simulink model "rlKinovaBallBalance_lags"  (R2024a)
settings: Solver=ode15s  StartTime=0.0  StopTime=inf  MaxStep=0.005  RelTol=1e-4  AbsTol=1e-4
values from neighbouring files (symbols this model uses):
  abs_max_torque_U = [6, 0.70, 2.12, 0.505]    [kinova_params.m]
  g = 3.71    [kinova_params.m]
  max_angular_vel = 2.0    (= 2)    [kinova_params.m]
  max_linear_vel = 0.6    [kinova_params.m]
  max_torque = [1.6; 0.6; 0.9; 0.5]    [kinova_params.m]
  max_torque_PD = [2.5; 0.6; 0.6; 0.3]    [kinova_params.m]
  R1_q0 = 0    [kinova_params.m]
  R2_q0 = deg2rad(20)    [kinova_params.m]
  R3_q0 = 0    [kinova_params.m]
  R4_q0 = deg2rad(135)    [kinova_params.m]
  R5_q0 = 0    [kinova_params.m]
  R6_q0 = deg2rad(-65)    [kinova_params.m]
  R7_q0 = deg2rad(-90)    [kinova_params.m]
  rlEpisodeFinalTime = 21    [kinova_params.m]
  rlStartTime = 0    [kinova_params.m]
  rlTimeStep = 0.01    [kinova_params.m]
  U0 = [-5.75, 0.10, -1.3, 0.0]    [kinova_params.m]
undefined symbols (not defined in the file or in its folder): Control, fluent0, L1, L2, L3, LS1, LS3, plate, R1, R2, R3, Rover, rover_path, RS1, RS3, Ts, vessel, X, Y, Z
libraries: sm_lib x251, nesl_utility x110, fl_lib x85, nesl_utility_internal x34, sdl_lib x20, simulink x16, ee_lib x10, mars_rover_lib x6, slpidlib x2, batteryecm_lib x2, robotalgslib x1, rllib x1
(part 1 of 13)
settings Model: VariantFading=off  Creator=cosorio  LastModifiedBy=dika
settings SolverCC: AlgebraicLoopSolver=TrustRegion  MaxZcPerStep=1
settings DataIOCC: DSMLogging=off
settings OptimizationCC: ReuseModelBlockBuffer=off
settings DebuggingCC: UnconnectedInputMsg=warning  UnconnectedOutputMsg=warning  UnconnectedLineMsg=warning
settings ModelReferenceCC: EnableRefExpFcnMdlSchedulingChecks=on
settings RTWCC: GPUComputeCapability=3.5  DLArmComputeVersion=19.05
settings ExplorerConfigSet: InternalSimMechanicsExplorerSettings="<ExplorerConfiguration><canonicalview>default</canonicalview><AnimationSetting><BasePlaybackSpeed>1.0</BasePlaybackSpeed><PlaybackSpeedFactor>1.0</PlaybackSpeedFactor></AnimationSetting><TilePanel><TileInfo><Tiles Columns=\"1\" Count=\"1\" Rows=\"1\"><Column Weight=\"1\"/><Row Weight=\"1\"/><Tile Height=\"1\" Width=\"1\" X=\"0\" Y=\"0\"/></Tiles></TileInfo><SceneInfo><SceneViewer><BGColor><R>1</R><G>1</G><B>1</B></BGColor><Camera><DoPerspective>off</DoPerspective><Position><X>0.835449044511457073</X><Y>-0.495506913595096854</Y><Z>0.970261214764596258</Z></Position><Center><X>0.258098775321831175</X><Y>0.0818433555945289881</Y><Z>0.392910945574970416</Z></Center><Up><X>-0.408248290463863073</X><Y>0.408248290463863073</Y><Z>0.816496580927726145</Z></Up><ViewLimDist>1</ViewLimDist><YLim>0.340419242978096004</YLim><XLim>0.488995507299471222</XLim></Camera></SceneViewer></SceneInfo></TilePanel><MechEditorPanel><Cameras/><GfxPanelCameraMap/><VideoCreator><PlaybackSpeedRatio>1.0</PlaybackSpeedRatio><FrameRate>30</FrameRate><VideoFormat>Motion JPEG AVI</VideoFormat><FrameSize>auto</FrameSize></VideoCreator></MechEditorPanel></ExplorerConfiguration>"

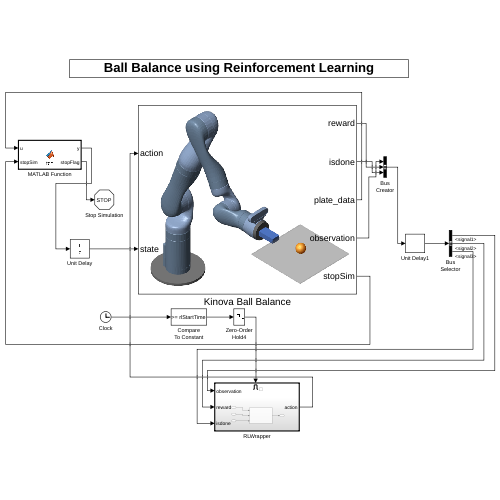
[thumbnail: Simulink's stored preview of the top-level diagram]
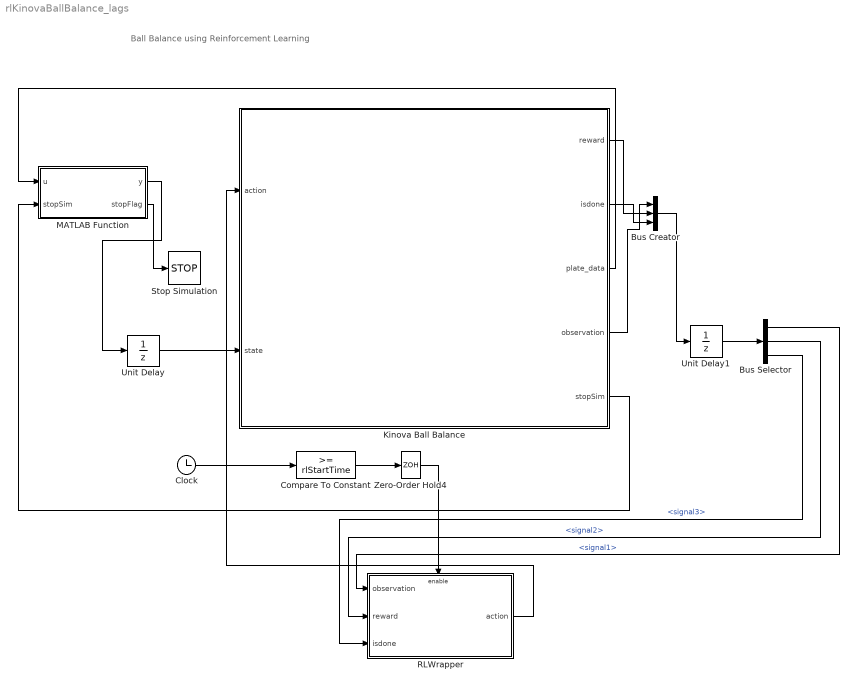
== system rlKinovaBallBalance_lags ==
  note: Ball Balance using Reinforcement Learning
  Bus Creator : BusCreator  Inputs=3
  Bus Selector : BusSelector  OutputSignals=signal1,signal2,signal3
  Clock : Clock
  Compare To Constant : simulink/Logic and Bit Operations/Compare To Constant  relop=>=  const=rlStartTime  OutDataTypeStr=boolean
  Kinova Ball Balance : Subsystem
      mask Display: image('$imagefile'); % Use "Edit Image" on toolstrip to change.
  MATLAB Function : MATLAB Function  TreatAsAtomicUnit=on
  RLWrapper : Subsystem  TreatAsAtomicUnit=on
  Stop Simulation : Stop
  Unit Delay : UnitDelay  SampleTime=-1  HasFrameUpgradeWarning=on
  Unit Delay1 : UnitDelay  SampleTime=-1  HasFrameUpgradeWarning=on
  Zero-Order Hold4 : ZeroOrderHold  SampleTime=Ts
  wires:
  MATLAB Function/1(y) -> Unit Delay/1
  Unit Delay/1 -> Kinova Ball Balance/2(state)
  Kinova Ball Balance/3(plate_data) -> MATLAB Function/1(u)
  Kinova Ball Balance/1(reward) -> Bus Creator/2
  Kinova Ball Balance/2(isdone) -> Bus Creator/3
  Bus Creator/1 -> Unit Delay1/1
  Unit Delay1/1 -> Bus Selector/1
  Kinova Ball Balance/4(observation) -> Bus Creator/1
  Bus Selector/2 -> RLWrapper/2(reward)  "<signal2>"
  Bus Selector/1 -> RLWrapper/1(observation)  "<signal1>"
  Bus Selector/3 -> RLWrapper/3(isdone)  "<signal3>"
  RLWrapper/1(action) -> Kinova Ball Balance/1(action)
  Compare To Constant/1 -> Zero-Order Hold4/1
  Clock/1 -> Compare To Constant/1
  Kinova Ball Balance/5(stopSim) -> MATLAB Function/2(stopSim)
  Zero-Order Hold4/1 -> RLWrapper/Enable
  MATLAB Function/2(stopFlag) -> Stop Simulation/1

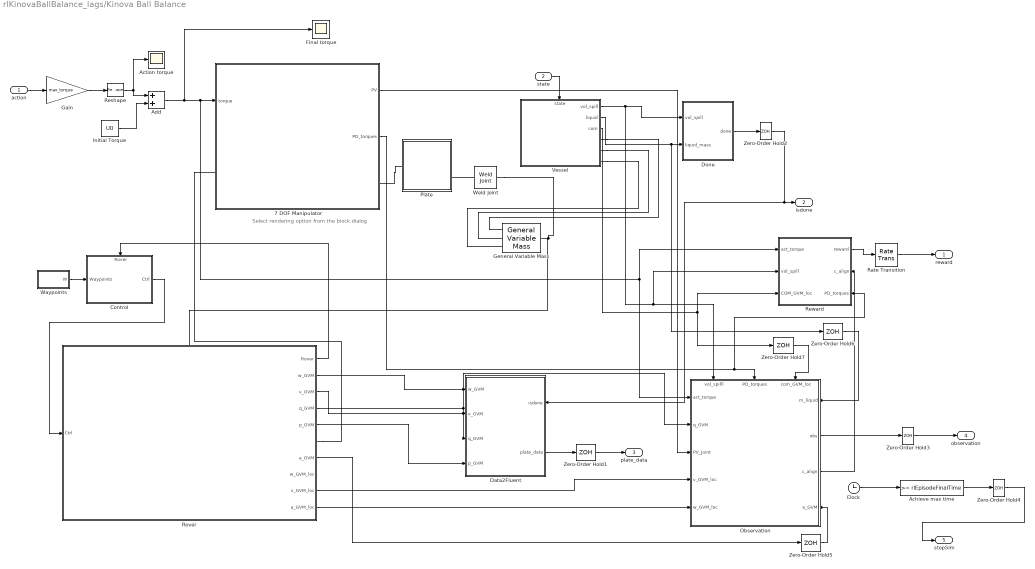
== system rlKinovaBallBalance_lags/Kinova Ball Balance ==
  note: Select rendering option from the block dialog
  action : Inport
  state : Inport  Port=2
  7 DOF Manipulator : Subsystem  mask{VChoice=3D Mesh}
      mask prompts: VChoice "Visualization"
      mask init:
      | choice = get_param(gcb,'VChoice');
      | vssBlk = bdroot + "/Kinova Ball Balance/7 DOF Manipulator" + ...
      |    ["/base_link/Base Link";
      |     "/Shoulder_Link/Shoulder Link";
      |     "/HalfArm1_Link/HalfArm1 Link";
      |     "/HalfArm2_Link/HalfArm2 Link";
      |     "/ForeArm_Link/ForeArm Link";
      |     "/Wrist1_Link/Wrist1 Link";
      |     "/Wrist2_Link/Wrist2 Link";
      |     "/Bracelet_Link/Bracelet Link"];
      | oldVariant = get_param(gcb,'LabelModeActiveChoice');
      | for ct = 1:numel(vssBlk)
      |     if strcmp(choice,'None')
      |         % turn off simscape visualization
      |         set_param(vssBlk(ct), 'LabelModeActiveChoice', 'Choice');
      |         set_param(bdroot, 'SimMechanicsOpenEditorOnUpdate', 'off');
      |     else
      |         % turn on simscape visualization
      |         set_param(vssBlk(ct), 'LabelModeActiveChoice', 'Choice_1');
      |         set_param(bdroot, 'SimMechanicsOpenEditorOnUpdate', 'on');
      |     end
      | end
      mask TypeOptions VChoice: None | 3D Mesh
      mask DialogControl DescGroupVar Prompt: Rendering
      mask DialogControl DescTextVar Prompt: Select options to visualize the robot. The 3D Mesh option requires the Robotics System Toolbox Robot Library Data support package.
      mask DialogControl ParameterGroupVar Prompt: Rendering options
      mask Display: image('$imagefile'); % Use "Edit Image" on toolstrip to change.
  Achieve max time : simulink/Logic and Bit Operations/Compare To Constant  relop=>=  const=rlEpisodeFinalTime  OutDataTypeStr=boolean
  Action torque : Scope
  Add : Sum
  Clock : Clock
  Control : Subsystem
      settings: PortSchema="{\"entries\":[{\"content\":{\"sides\":[{\"content\":{\"connectorIds\":[\"In1\"]},\"type\":\"ConnectorPlacement.EquallySpacedRectSide\",\"uuid\":\"c3d7e194-f80c-4e55-926d-d58bd075eaae\"},{\"content\":{\"connectorIds\":[\"Out1\"],\"side\":\"RIGHT\"},\"type\":\"ConnectorPlacement.EquallySpacedRectSide\",\"uuid\":\"f7d0fe5b-9aee-419d-9958-60715756a35f\"},{\"content\":{\"connectorIds\":[\"In2\"],\"side\":\"TOP\"},\"type\":\"ConnectorPlacement.EquallySpacedRectSide\",\"uuid\":\"f91288f6-db9b-4528-8971-65b8d23b6b9e\"},{\"content\":{\"side\":\"BOTTOM\"},\"type\":\"ConnectorPlacement.EquallySpacedRectSide\",\"uuid\":\"aa6c6625-5d2c-4cfa-81dd-42b85ff12eb6\"}]},\"type\":\"ConnectorPlacement.EquallySpacedConnector\",\"uuid\":\"3d017957-8f60-4a25-bb87-fd20ede06be0\"}],\"packageUris\":[\"http://schema.mathworks.com/mf0/Connector/R2020b\"],\"version\":\"1.0\"}"
  Data2Fluent : Subsystem
      settings: PortSchema="{\"entries\":[{\"content\":{\"sides\":[{\"content\":{\"connectorIds\":[\"In1\",\"In2\",\"In3\",\"In4\"]},\"type\":\"ConnectorPlacement.EquallySpacedRectSide\",\"uuid\":\"d2580b95-1100-4ac1-85be-11deaa0122b6\"},{\"content\":{\"connectorIds\":[\"In5\",\"Out1\"],\"side\":\"RIGHT\"},\"type\":\"ConnectorPlacement.EquallySpacedRectSide\",\"uuid\":\"70e7c1d6-5559-4655-a09c-42417fa5168e\"},{\"content\":{\"side\":\"TOP\"},\"type\":\"ConnectorPlacement.EquallySpacedRectSide\",\"uuid\":\"be848a5e-034e-48a0-9929-21b8a0be8f3f\"}]},\"type\":\"ConnectorPlacement.EquallySpacedConnector\",\"uuid\":\"450ed5cd-5d65-4ed6-b2f4-ea103b2a194f\"}],\"packageUris\":[\"http://schema.mathworks.com/mf0/Connector/R2020b\"],\"version\":\"1.0\"}"
  Done : Subsystem
  Final torque : Scope
  Gain : Gain  Gain=max_torque
  General Variable Mass : sm_lib/Body Elements/Variable Mass/General Variable Mass  VariableInertiaType=Custom  MassType=TimeVarying  Mass=1  MassUnits=kg  CenterOfMassType=TimeVarying  CenterOfMass=[0 0 0]  CenterOfMassUnits=m  InertiaMatrixType=TimeVarying  MomentsOfInertia=[1 1 1]  MomentsOfInertiaUnits=kg*m^2  ProductsOfInertia=[0 0 0]  ProductsOfInertiaUnits=kg*m^2  GraphicType=Marker  MarkerShape=Sphere  MarkerSize=100  GraphicVisPropType=SimpleVisualProperties  GraphicDiffuseColor=[0.5 0.5 0.5]  GraphicOpacity=1  GraphicSpecularColor=[0.5 0.5 0.5 1.0]  GraphicAmbientColor=[0.15 0.15 0.15 1.0]  GraphicEmissiveColor=[0.0 0.0 0.0 1.0]  GraphicShininess=75
  Initial Torque : Constant  Value=U0
  Observation : Subsystem
      settings: PortSchema="{\"entries\":[{\"content\":{\"sides\":[{\"content\":{\"connectorIds\":[\"In1\",\"In2\",\"In3\",\"In4\",\"In5\"]},\"type\":\"ConnectorPlacement.EquallySpacedRectSide\",\"uuid\":\"1f819b26-4f65-41ef-a298-effbe2270ef5\"},{\"content\":{\"connectorIds\":[\"In9\",\"Out1\",\"Out2\",\"In10\"],\"side\":\"RIGHT\"},\"type\":\"ConnectorPlacement.EquallySpacedRectSide\",\"uuid\":\"491918ce-fc7c-4684-8246-c6be896d1069\"},{\"content\":{\"connectorIds\":[\"In6\",\"In7\",\"In8\"],\"side\":\"TOP\"},\"type\":\"ConnectorPlacement.EquallySpacedRectSide\",\"uuid\":\"2c72369d-314e-4a7a-93e9-42ede2c72e3e\"},{\"content\":{\"side\":\"BOTTOM\"},\"type\":\"ConnectorPlacement.EquallySpacedRectSide\",\"uuid\":\"f3733c5f-ece3-4511-b18e-584e8db17e04\"}]},\"type\":\"ConnectorPlacement.EquallySpacedConnector\",\"uuid\":\"9fa8ee02-96e6-4ca3-a042-fc1037b88a21\"}],\"packageUris\":[\"http://schema.mathworks.com/mf0/Connector/R2020b\"],\"version\":\"1.0\"}"
  Plate : Subsystem
      mask Display: image('$imagefile'); % Use "Edit Image" on toolstrip to change.
  Rate Transition : RateTransition  OutPortSampleTime=Ts
  Reshape : Reshape  OutputDimensionality=Row vector (2-D)
  Reward : Subsystem
      settings: PortSchema="{\"entries\":[{\"content\":{\"sides\":[{\"content\":{\"connectorIds\":[\"In1\",\"In2\",\"In3\"]},\"type\":\"ConnectorPlacement.EquallySpacedRectSide\",\"uuid\":\"5d933a9d-95d3-47ea-9901-687451c9fbea\"},{\"content\":{\"connectorIds\":[\"Out1\",\"In4\",\"In5\"],\"side\":\"RIGHT\"},\"type\":\"ConnectorPlacement.EquallySpacedRectSide\",\"uuid\":\"29a52886-19a3-4b66-bd74-438fafa7a07e\"},{\"content\":{\"side\":\"TOP\"},\"type\":\"ConnectorPlacement.EquallySpacedRectSide\",\"uuid\":\"3fc8db25-df22-4142-aace-f1d33f79f87b\"}]},\"type\":\"ConnectorPlacement.EquallySpacedConnector\",\"uuid\":\"35028655-dfec-48a2-9708-f2ca1e0329cc\"}],\"packageUris\":[\"http://schema.mathworks.com/mf0/Connector/R2020b\"],\"version\":\"1.0\"}"
  Rover : Subsystem
      settings: PortSchema="{\"entries\":[{\"content\":{\"sides\":[{\"content\":{\"connectorIds\":[\"In1\"]},\"type\":\"ConnectorPlacement.EquallySpacedRectSide\",\"uuid\":\"f99998cd-7f44-4958-986a-883545f054e6\"},{\"content\":{\"connectorIds\":[\"Out1\",\"Out2\",\"Out3\",\"Out4\",\"Out5\",\"RConn1\",\"Out6\",\"Out7\",\"Out8\",\"Out9\"],\"side\":\"RIGHT\"},\"type\":\"ConnectorPlacement.EquallySpacedRectSide\",\"uuid\":\"f32f7cef-c0c0-4695-a0b9-122721d5e398\"},{\"content\":{\"connectorIds\":[\"LConn1\"],\"side\":\"TOP\"},\"type\":\"ConnectorPlacement.EquallySpacedRectSide\",\"uuid\":\"7344a25a-a782-4a10-9f2c-7810aaabe583\"}]},\"type\":\"ConnectorPlacement.EquallySpacedConnector\",\"uuid\":\"21be1294-6a1a-40f2-9693-1f444d473d1d\"}],\"packageUris\":[\"http://schema.mathworks.com/mf0/Connector/R2020b\"],\"version\":\"1.0\"}"
      mask Display: image('mars_rover_terrain_chassis.png');
  Vessel : Subsystem
      settings: PortSchema="{\"entries\":[{\"content\":{\"sides\":[{\"content\":{},\"type\":\"ConnectorPlacement.EquallySpacedRectSide\",\"uuid\":\"dcdc7885-492c-498f-a442-6424ac696a17\"},{\"content\":{\"connectorIds\":[\"Out1\",\"Out2\",\"Out3\",\"RConn1\",\"RConn2\",\"RConn3\"],\"side\":\"RIGHT\"},\"type\":\"ConnectorPlacement.EquallySpacedRectSide\",\"uuid\":\"323b1566-cd85-443c-b64d-37bc7cbbf4f4\"},{\"content\":{\"connectorIds\":[\"In1\"],\"side\":\"TOP\"},\"type\":\"ConnectorPlacement.EquallySpacedRectSide\",\"uuid\":\"18ea813b-2836-4610-9c93-f73d3123e495\"},{\"content\":{\"side\":\"BOTTOM\"},\"type\":\"ConnectorPlacement.EquallySpacedRectSide\",\"uuid\":\"bc1a7a95-2321-49a3-b611-36fcfe7a8e53\"}]},\"type\":\"ConnectorPlacement.EquallySpacedConnector\",\"uuid\":\"32ac73cf-4f09-4885-b08e-9ed6f73651df\"}],\"packageUris\":[\"http://schema.mathworks.com/mf0/Connector/R2020b\"],\"version\":\"1.0\"}"
  Waypoints : Subsystem
      mask Display:
      | px = evalin('base','rover_path.x');
      | py = evalin('base','rover_path.y');
      | plot(px,py)
  Weld Joint : sm_lib/Joints/Weld Joint  JointMode=Normal  CompositeWrenchDir=FollowerOnBase  CompositeWrenchFrame=BaseFrame  SenseConstraintForce=off  SenseConstraintTorque=off  SenseTotalForce=off  SenseTotalTorque=off
  Zero-Order Hold{1..7} (7 alike) : ZeroOrderHold  SampleTime=Ts
  reward : Outport
  isdone : Outport  Port=2
  plate_data : Outport  Port=3
  observation : Outport  Port=4
  stopSim : Outport  Port=5
  wires:
  state/1 -> Vessel/1(state)
  7 DOF Manipulator/1(PV) -> Observation/3(PV_Joint)
  Zero-Order Hold1/1 -> plate_data/1
  Waypoints/1(W) -> Control/1(Waypoints)
  Control/1(Ctrl) -> Rover/1(Ctrl)
  Rover/1(Rover) -> Control/2(Rover)
  Reward/1(reward) -> Rate Transition/1
  Data2Fluent/1(plate_data) -> Zero-Order Hold1/1
  Observation/1(obs) -> Zero-Order Hold3/1
  Rate Transition/1 -> reward/1
  action/1 -> Gain/1
  Done/1(done) -> Zero-Order Hold2/1
  Zero-Order Hold2/1 -> isdone/1, Data2Fluent/5(isdone)
  Gain/1 -> Reshape/1
  Reshape/1 -> Add/1, Action torque/1
  Initial Torque/1 -> Add/2
  Vessel/3(com) -> Zero-Order Hold7/1, Reward/3(COM_GVM_loc)
  Zero-Order Hold3/1 -> observation/1
  Rover/5(p_GVM) -> Data2Fluent/4(p_GVM)
  Rover/4(q_GVM) -> Data2Fluent/3(q_GVM), Observation/2(q_GVM)
  Rover/3(v_GVM) -> Data2Fluent/2(v_GVM)
  Rover/2(w_GVM) -> Data2Fluent/1(w_GVM)
  Vessel/2(liquid) -> Zero-Order Hold6/1, Done/2(liquid_mass)
  Vessel/1(vol_spill) -> Reward/2(vol_spill), Observation/6(vol_spilll), Done/1(vol_spill)
  Clock/1 -> Achieve max time/1
  Achieve max time/1 -> Zero-Order Hold4/1
  Zero-Order Hold4/1 -> stopSim/1
  Rover/6(a_GVM) -> Zero-Order Hold5/1
  Zero-Order Hold5/1 -> Observation/10(a_GVM)
  Zero-Order Hold6/1 -> Observation/9(m_liquid)
  Zero-Order Hold7/1 -> Observation/8(com_GVM_loc)
  Observation/2(c_align) -> Reward/4(c_align)
  Add/1 -> Final torque/1, Observation/1(act_torque), Reward/1(act_torque), 7 DOF Manipulator/1(torque)
  7 DOF Manipulator/2(PD_torques) -> Reward/5(PD_torques), Observation/7(PD_torques)
  Rover/8(v_GVM_loc) -> Observation/4(v_GVM_loc)
  Rover/9(a_GVM_loc) -> Observation/5(w_GVM_loc)
  connections:
  Rover/RConn1 -- 7 DOF Manipulator/LConn1
  Vessel/RConn3 -- General Variable Mass/LConn3
  Weld Joint/RConn1 -- Rover/LConn1 -- General Variable Mass/RConn1
  Vessel/RConn2 -- General Variable Mass/LConn2
  Vessel/RConn1 -- General Variable Mass/LConn1
  Weld Joint/LConn1 -- Plate/LConn2
  7 DOF Manipulator/RConn1 -- Plate/RConn1

== system rlKinovaBallBalance_lags/RLWrapper ==
  observation : Inport
  reward : Inport  Port=2
  isdone : Inport  Port=3
  Enable : EnablePort
  RL Agent : rllib/RL Agent  Agent=agentObj  ExternalActionAsInput=off  ProvideLastAction=off  ProvideCumRwd=off  TreatAsDirectFeedthrough=on  UseStrictObservationDataTypes=off
  action : Outport
  wires:
  isdone/1 -> RL Agent/3
  observation/1 -> RL Agent/1
  reward/1 -> RL Agent/2
  RL Agent/1 -> action/1

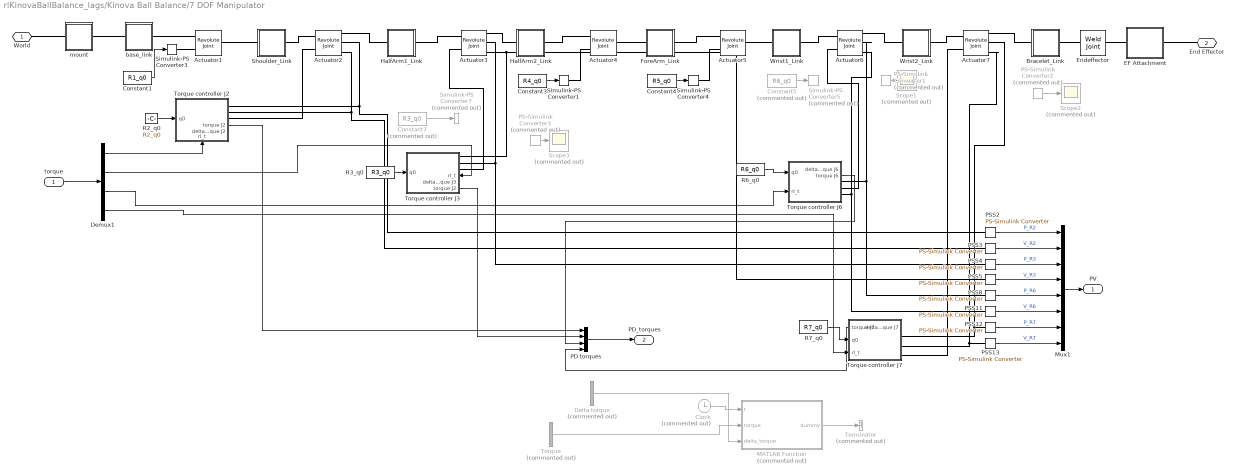
== system rlKinovaBallBalance_lags/Kinova Ball Balance/7 DOF Manipulator ==
  torque : Inport
  Actuator1 : sm_lib/Joints/Revolute Joint  JointMode=Normal  CompositeWrenchDir=FollowerOnBase  CompositeWrenchFrame=BaseFrame  SenseConstraintForce=off  SenseConstraintTorque=off  SenseTotalForce=off  SenseTotalTorque=off  PositionTargetSpecify=on  PositionTargetPriority=High  PositionTargetValue=R1_q0  PositionTargetValueUnits=rad  VelocityTargetSpecify=off  VelocityTargetPriority=High  VelocityTargetValue=0  VelocityTargetValueUnits=deg/s  EquilibriumPosition=0  EquilibriumPositionUnits=deg  SpringStiffness=0  SpringStiffnessUnits=N*m/deg  DampingCoefficient=0  DampingCoefficientUnits=m^2*kg/s/rad  LowerLimitSpecify=off  LowerLimitBound=-90  LowerLimitBoundUnits=deg  LowerLimitStiffness=1e4  LowerLimitStiffnessUnits=N*m/deg  LowerLimitDamping=10  LowerLimitDampingUnits=N*m/(deg/s)  LowerLimitTransitionRegionWidth=0.1  LowerLimitTransitionRegionWidthUnits=deg  UpperLimitSpecify=off  UpperLimitBound=90  UpperLimitBoundUnits=deg  UpperLimitStiffness=1e4  UpperLimitStiffnessUnits=N*m/deg  UpperLimitDamping=10  UpperLimitDampingUnits=N*m/(deg/s)  UpperLimitTransitionRegionWidth=0.1  UpperLimitTransitionRegionWidthUnits=deg  TorqueActuationMode=ComputedTorque  MotionActuationMode=InputMotion  SensePosition=off  SenseVelocity=off  SenseAcceleration=off  SenseTorqueForce=off  SenseLowerLimitTorqueForce=off  SenseUpperLimitTorqueForce=off
  Actuator2 : sm_lib/Joints/Revolute Joint  JointMode=Normal  CompositeWrenchDir=FollowerOnBase  CompositeWrenchFrame=BaseFrame  SenseConstraintForce=off  SenseConstraintTorque=off  SenseTotalForce=off  SenseTotalTorque=off  PositionTargetSpecify=on  PositionTargetPriority=High  PositionTargetValue=R2_q0  PositionTargetValueUnits=rad  VelocityTargetSpecify=off  VelocityTargetPriority=High  VelocityTargetValue=0  VelocityTargetValueUnits=deg/s  EquilibriumPosition=0  EquilibriumPositionUnits=deg  SpringStiffness=50  SpringStiffnessUnits=N*m/rad  DampingCoefficient=5  DampingCoefficientUnits=N*m*s/rad  LowerLimitSpecify=on  LowerLimitBound=-2.2  LowerLimitBoundUnits=rad  LowerLimitStiffness=1e4  LowerLimitStiffnessUnits=N*m/deg  LowerLimitDamping=10  LowerLimitDampingUnits=N*m/(deg/s)  LowerLimitTransitionRegionWidth=0.1  LowerLimitTransitionRegionWidthUnits=deg  UpperLimitSpecify=on  UpperLimitBound=2.2  UpperLimitBoundUnits=rad  UpperLimitStiffness=1e4  UpperLimitStiffnessUnits=N*m/deg  UpperLimitDamping=10  UpperLimitDampingUnits=N*m/(deg/s)  UpperLimitTransitionRegionWidth=0.1  UpperLimitTransitionRegionWidthUnits=deg  TorqueActuationMode=InputTorque  MotionActuationMode=ComputedMotion  SensePosition=on  SenseVelocity=on  SenseAcceleration=off  SenseTorqueForce=off  SenseLowerLimitTorqueForce=off  SenseUpperLimitTorqueForce=off
  Actuator3 : sm_lib/Joints/Revolute Joint  JointMode=Normal  CompositeWrenchDir=FollowerOnBase  CompositeWrenchFrame=BaseFrame  SenseConstraintForce=off  SenseConstraintTorque=off  SenseTotalForce=off  SenseTotalTorque=off  PositionTargetSpecify=on  PositionTargetPriority=High  PositionTargetValue=R3_q0  PositionTargetValueUnits=rad  VelocityTargetSpecify=off  VelocityTargetPriority=High  VelocityTargetValue=0  VelocityTargetValueUnits=deg/s  EquilibriumPosition=0  EquilibriumPositionUnits=deg  SpringStiffness=50  SpringStiffnessUnits=N*m/rad  DampingCoefficient=5  DampingCoefficientUnits=N*m*s/rad  LowerLimitSpecify=off  LowerLimitBound=-90  LowerLimitBoundUnits=deg  LowerLimitStiffness=1e4  LowerLimitStiffnessUnits=N*m/deg  LowerLimitDamping=10  LowerLimitDampingUnits=N*m/(deg/s)  LowerLimitTransitionRegionWidth=0.1  LowerLimitTransitionRegionWidthUnits=deg  UpperLimitSpecify=off  UpperLimitBound=90  UpperLimitBoundUnits=deg  UpperLimitStiffness=1e4  UpperLimitStiffnessUnits=N*m/deg  UpperLimitDamping=10  UpperLimitDampingUnits=N*m/(deg/s)  UpperLimitTransitionRegionWidth=0.1  UpperLimitTransitionRegionWidthUnits=deg  TorqueActuationMode=InputTorque  MotionActuationMode=ComputedMotion  SensePosition=on  SenseVelocity=on  SenseAcceleration=off  SenseTorqueForce=off  SenseLowerLimitTorqueForce=off  SenseUpperLimitTorqueForce=off
  Actuator4 : sm_lib/Joints/Revolute Joint  JointMode=Normal  CompositeWrenchDir=FollowerOnBase  CompositeWrenchFrame=BaseFrame  SenseConstraintForce=off  SenseConstraintTorque=off  SenseTotalForce=off  SenseTotalTorque=off  PositionTargetSpecify=on  PositionTargetPriority=High  PositionTargetValue=R4_q0  PositionTargetValueUnits=rad  VelocityTargetSpecify=off  VelocityTargetPriority=High  VelocityTargetValue=0  VelocityTargetValueUnits=deg/s  EquilibriumPosition=0  EquilibriumPositionUnits=deg  SpringStiffness=0  SpringStiffnessUnits=N*m/deg  DampingCoefficient=0  DampingCoefficientUnits=m^2*kg/s/rad  LowerLimitSpecify=on  LowerLimitBound=-2.5656  LowerLimitBoundUnits=rad  LowerLimitStiffness=1e4  LowerLimitStiffnessUnits=N*m/deg  LowerLimitDamping=10  LowerLimitDampingUnits=N*m/(deg/s)  LowerLimitTransitionRegionWidth=0.1  LowerLimitTransitionRegionWidthUnits=deg  UpperLimitSpecify=on  UpperLimitBound=2.5656  UpperLimitBoundUnits=rad  UpperLimitStiffness=1e4  UpperLimitStiffnessUnits=N*m/deg  UpperLimitDamping=10  UpperLimitDampingUnits=N*m/(deg/s)  UpperLimitTransitionRegionWidth=0.1  UpperLimitTransitionRegionWidthUnits=deg  TorqueActuationMode=ComputedTorque  MotionActuationMode=InputMotion  SensePosition=off  SenseVelocity=off  SenseAcceleration=off  SenseTorqueForce=off  SenseLowerLimitTorqueForce=off  SenseUpperLimitTorqueForce=off
  Actuator5 : sm_lib/Joints/Revolute Joint  JointMode=Normal  CompositeWrenchDir=FollowerOnBase  CompositeWrenchFrame=BaseFrame  SenseConstraintForce=off  SenseConstraintTorque=off  SenseTotalForce=off  SenseTotalTorque=off  PositionTargetSpecify=on  PositionTargetPriority=High  PositionTargetValue=R5_q0  PositionTargetValueUnits=rad  VelocityTargetSpecify=off  VelocityTargetPriority=High  VelocityTargetValue=0  VelocityTargetValueUnits=deg/s  EquilibriumPosition=0  EquilibriumPositionUnits=deg  SpringStiffness=0  SpringStiffnessUnits=N*m/deg  DampingCoefficient=0  DampingCoefficientUnits=m^2*kg/s/rad  LowerLimitSpecify=off  LowerLimitBound=-90  LowerLimitBoundUnits=deg  LowerLimitStiffness=1e4  LowerLimitStiffnessUnits=N*m/deg  LowerLimitDamping=10  LowerLimitDampingUnits=N*m/(deg/s)  LowerLimitTransitionRegionWidth=0.1  LowerLimitTransitionRegionWidthUnits=deg  UpperLimitSpecify=off  UpperLimitBound=90  UpperLimitBoundUnits=deg  UpperLimitStiffness=1e4  UpperLimitStiffnessUnits=N*m/deg  UpperLimitDamping=10  UpperLimitDampingUnits=N*m/(deg/s)  UpperLimitTransitionRegionWidth=0.1  UpperLimitTransitionRegionWidthUnits=deg  TorqueActuationMode=ComputedTorque  MotionActuationMode=InputMotion  SensePosition=off  SenseVelocity=off  SenseAcceleration=off  SenseTorqueForce=off  SenseLowerLimitTorqueForce=off  SenseUpperLimitTorqueForce=off
  Actuator6 : sm_lib/Joints/Revolute Joint  JointMode=Normal  CompositeWrenchDir=FollowerOnBase  CompositeWrenchFrame=BaseFrame  SenseConstraintForce=off  SenseConstraintTorque=off  SenseTotalForce=off  SenseTotalTorque=off  PositionTargetSpecify=on  PositionTargetPriority=High  PositionTargetValue=R6_q0  PositionTargetValueUnits=rad  VelocityTargetSpecify=off  VelocityTargetPriority=High  VelocityTargetValue=0  VelocityTargetValueUnits=deg/s  EquilibriumPosition=0  EquilibriumPositionUnits=deg  SpringStiffness=0  SpringStiffnessUnits=N*m/deg  DampingCoefficient=0  DampingCoefficientUnits=m^2*kg/s/rad  LowerLimitSpecify=on  LowerLimitBound=-2.05  LowerLimitBoundUnits=rad  LowerLimitStiffness=1e4  LowerLimitStiffnessUnits=N*m/deg  LowerLimitDamping=10  LowerLimitDampingUnits=N*m/(deg/s)  LowerLimitTransitionRegionWidth=0.1  LowerLimitTransitionRegionWidthUnits=deg  UpperLimitSpecify=on  UpperLimitBound=2.05  UpperLimitBoundUnits=rad  UpperLimitStiffness=1e4  UpperLimitStiffnessUnits=N*m/deg  UpperLimitDamping=10  UpperLimitDampingUnits=N*m/(deg/s)  UpperLimitTransitionRegionWidth=0.1  UpperLimitTransitionRegionWidthUnits=deg  TorqueActuationMode=InputTorque  MotionActuationMode=ComputedMotion  SensePosition=on  SenseVelocity=on  SenseAcceleration=off  SenseTorqueForce=off  SenseLowerLimitTorqueForce=off  SenseUpperLimitTorqueForce=off
  Actuator7 : sm_lib/Joints/Revolute Joint  JointMode=Normal  CompositeWrenchDir=FollowerOnBase  CompositeWrenchFrame=BaseFrame  SenseConstraintForce=off  SenseConstraintTorque=off  SenseTotalForce=off  SenseTotalTorque=off  PositionTargetSpecify=on  PositionTargetPriority=High  PositionTargetValue=R7_q0  PositionTargetValueUnits=rad  VelocityTargetSpecify=off  VelocityTargetPriority=High  VelocityTargetValue=0  VelocityTargetValueUnits=deg/s  EquilibriumPosition=0  EquilibriumPositionUnits=deg  SpringStiffness=0  SpringStiffnessUnits=N*m/deg  DampingCoefficient=0  DampingCoefficientUnits=m^2*kg/s/rad  LowerLimitSpecify=off  LowerLimitBound=-90  LowerLimitBoundUnits=deg  LowerLimitStiffness=1e4  LowerLimitStiffnessUnits=N*m/deg  LowerLimitDamping=10  LowerLimitDampingUnits=N*m/(deg/s)  LowerLimitTransitionRegionWidth=0.1  LowerLimitTransitionRegionWidthUnits=deg  UpperLimitSpecify=off  UpperLimitBound=90  UpperLimitBoundUnits=deg  UpperLimitStiffness=1e4  UpperLimitStiffnessUnits=N*m/deg  UpperLimitDamping=10  UpperLimitDampingUnits=N*m/(deg/s)  UpperLimitTransitionRegionWidth=0.1  UpperLimitTransitionRegionWidthUnits=deg  TorqueActuationMode=InputTorque  MotionActuationMode=ComputedMotion  SensePosition=on  SenseVelocity=on  SenseAcceleration=off  SenseTorqueForce=off  SenseLowerLimitTorqueForce=off  SenseUpperLimitTorqueForce=off
  Bracelet_Link : Subsystem
  Clock : Clock  Commented=on
  Constant1 : Constant  Value=R1_q0
  Constant3 : Constant  Value=R4_q0
  Constant4 : Constant  Value=R5_q0
  Constant5 : Constant  Commented=on  Value=R6_q0
  Constant7 : Constant  Commented=on  Value=R3_q0
  Delta torque : Mux  Commented=on
  Demux1 : Demux
  EF Attachment : Subsystem
  Endeffector : sm_lib/Joints/Weld Joint  JointMode=Normal  CompositeWrenchDir=FollowerOnBase  CompositeWrenchFrame=BaseFrame  SenseConstraintForce=off  SenseConstraintTorque=off  SenseTotalForce=off  SenseTotalTorque=off
  ForeArm_Link : Subsystem
  HalfArm1_Link : Subsystem
  HalfArm2_Link : Subsystem
  MATLAB Function : MATLAB Function  Commented=on  TreatAsAtomicUnit=on
  Mux1 : Mux  Inputs=8
  PD torques : Mux
  PS-Simulink Converter1 : nesl_utility/PS-Simulink Converter  Commented=on  PhysicalDomain=network_engine_domain  SubClassName=ps_output  LeftPortType=input  RightPortType=output  PseudoPeriodic=off  Frequencies=[]  VectorFormat=inherit  Unit=inherit  AffineConversion=off
  PS-Simulink Converter2 : nesl_utility/PS-Simulink Converter  Commented=on  PhysicalDomain=network_engine_domain  SubClassName=ps_output  LeftPortType=input  RightPortType=output  PseudoPeriodic=off  Frequencies=[]  VectorFormat=inherit  Unit=inherit  AffineConversion=off
  PS-Simulink Converter3 : nesl_utility/PS-Simulink Converter  Commented=on  PhysicalDomain=network_engine_domain  SubClassName=ps_output  LeftPortType=input  RightPortType=output  PseudoPeriodic=off  Frequencies=[]  VectorFormat=inherit  Unit=inherit  AffineConversion=off
  PSS{3,5,11,13} (4 alike) : nesl_utility_internal/PS-Simulink Converter  PhysicalDomain=network_engine_domain  SubClassName=ps_output  LeftPortType=input  RightPortType=output  PseudoPeriodic=off  Frequencies=[]  VectorFormat=1-D array  Unit=rad/s  AffineConversion=off
  PSS{2,4,8,12} (4 alike) : nesl_utility_internal/PS-Simulink Converter  PhysicalDomain=network_engine_domain  SubClassName=ps_output  LeftPortType=input  RightPortType=output  PseudoPeriodic=off  Frequencies=[]  VectorFormat=1-D array  Unit=rad  AffineConversion=off
  R2_q0 : Constant  Value=R2_q0
  R3_q0 : Constant  Value=R3_q0
  R6_q0 : Constant  Value=R6_q0
  R7_q0 : Constant  Value=R7_q0
  Scope1 : Scope  Commented=on
  Scope2 : Scope  Commented=on
  Scope3 : Scope  Commented=on
  Shoulder_Link : Subsystem
  Simulink-PS Converter1 : nesl_utility_internal/Simulink-PS Converter  PhysicalDomain=network_engine_domain  SubClassName=ps_input  LeftPortType=input  RightPortType=output  PseudoPeriodic=off  Frequencies=[]  NoiseDistribution=none  NoiseParameters=[]  Unit=1  AffineConversion=off  FilteringAndDerivatives=provide  SimscapeFilterOrder=1  InputFilterTimeConstant=0.001  UdotUserProvided=0
  Simulink-PS Converter3 : nesl_utility_internal/Simulink-PS Converter  PhysicalDomain=network_engine_domain  SubClassName=ps_input  LeftPortType=input  RightPortType=output  PseudoPeriodic=off  Frequencies=[]  NoiseDistribution=none  NoiseParameters=[]  Unit=1  AffineConversion=off  FilteringAndDerivatives=provide  SimscapeFilterOrder=1  InputFilterTimeConstant=0.001  UdotUserProvided=0
  Simulink-PS Converter4 : nesl_utility_internal/Simulink-PS Converter  PhysicalDomain=network_engine_domain  SubClassName=ps_input  LeftPortType=input  RightPortType=output  PseudoPeriodic=off  Frequencies=[]  NoiseDistribution=none  NoiseParameters=[]  Unit=1  AffineConversion=off  FilteringAndDerivatives=provide  SimscapeFilterOrder=1  InputFilterTimeConstant=0.001  UdotUserProvided=0
  Simulink-PS Converter5 : nesl_utility_internal/Simulink-PS Converter  Commented=on  PhysicalDomain=network_engine_domain  SubClassName=ps_input  LeftPortType=input  RightPortType=output  PseudoPeriodic=off  Frequencies=[]  NoiseDistribution=none  NoiseParameters=[]  Unit=1  AffineConversion=off  FilteringAndDerivatives=provide  SimscapeFilterOrder=1  InputFilterTimeConstant=0.001  UdotUserProvided=0
  Simulink-PS Converter7 : nesl_utility_internal/Simulink-PS Converter  Commented=on  PhysicalDomain=network_engine_domain  SubClassName=ps_input  LeftPortType=input  RightPortType=output  PseudoPeriodic=off  Frequencies=[]  NoiseDistribution=none  NoiseParameters=[]  Unit=1  AffineConversion=off  FilteringAndDerivatives=provide  SimscapeFilterOrder=1  InputFilterTimeConstant=0.001  UdotUserProvided=0
  Terminator : Terminator  Commented=on
  Torque : Mux  Commented=on
  Torque controller J2 : Subsystem
      settings: PortSchema="{\"entries\":[{\"content\":{\"sides\":[{\"content\":{\"connectorIds\":[\"In1\"]},\"type\":\"ConnectorPlacement.EquallySpacedRectSide\",\"uuid\":\"095988aa-34ff-41fa-a977-f46d39e23b2a\"},{\"content\":{\"connectorIds\":[\"RConn1\",\"RConn2\",\"RConn3\",\"Out1\",\"Out2\"],\"side\":\"RIGHT\"},\"type\":\"ConnectorPlacement.EquallySpacedRectSide\",\"uuid\":\"f68620a5-2921-48f0-865e-8506c5ca8f7b\"},{\"content\":{\"side\":\"TOP\"},\"type\":\"ConnectorPlacement.EquallySpacedRectSide\",\"uuid\":\"eeebf0d3-0cb1-47e5-8559-57fe666debe6\"},{\"content\":{\"connectorIds\":[\"In2\"],\"side\":\"BOTTOM\"},\"type\":\"ConnectorPlacement.EquallySpacedRectSide\",\"uuid\":\"535c76d7-2393-4bc1-beaf-0c16d2a56ade\"}]},\"type\":\"ConnectorPlacement.EquallySpacedConnector\",\"uuid\":\"bdca3cdb-44ac-4f4f-9fc0-a63e5a64f5ef\"}],\"packageUris\":[\"http://schema.mathworks.com/mf0/Connector/R2020b\"],\"version\":\"1.0\"}"
  Torque controller J3 : Subsystem
      settings: PortSchema="{\"entries\":[{\"content\":{\"sides\":[{\"content\":{\"connectorIds\":[\"In1\"]},\"type\":\"ConnectorPlacement.EquallySpacedRectSide\",\"uuid\":\"095988aa-34ff-41fa-a977-f46d39e23b2a\"},{\"content\":{\"connectorIds\":[\"RConn1\",\"RConn2\",\"RConn3\",\"In2\",\"Out1\",\"Out2\"],\"side\":\"RIGHT\"},\"type\":\"ConnectorPlacement.EquallySpacedRectSide\",\"uuid\":\"f68620a5-2921-48f0-865e-8506c5ca8f7b\"},{\"content\":{\"side\":\"TOP\"},\"type\":\"ConnectorPlacement.EquallySpacedRectSide\",\"uuid\":\"eeebf0d3-0cb1-47e5-8559-57fe666debe6\"}]},\"type\":\"ConnectorPlacement.EquallySpacedConnector\",\"uuid\":\"bdca3cdb-44ac-4f4f-9fc0-a63e5a64f5ef\"}],\"packageUris\":[\"http://schema.mathworks.com/mf0/Connector/R2020b\"],\"version\":\"1.0\"}"
  Torque controller J6 : Subsystem
  Torque controller J7 : Subsystem
      settings: PortSchema="{\"entries\":[{\"content\":{\"sides\":[{\"content\":{\"connectorIds\":[\"Out2\",\"In1\",\"In2\"]},\"type\":\"ConnectorPlacement.EquallySpacedRectSide\",\"uuid\":\"2ba4fbae-ef3a-4af5-8190-ba61f5af81f4\"},{\"content\":{\"connectorIds\":[\"Out1\",\"RConn1\",\"RConn2\",\"RConn3\"],\"side\":\"RIGHT\"},\"type\":\"ConnectorPlacement.EquallySpacedRectSide\",\"uuid\":\"932be769-d022-4bca-b733-10e6d8a94a22\"},{\"content\":{\"side\":\"TOP\"},\"type\":\"ConnectorPlacement.EquallySpacedRectSide\",\"uuid\":\"afed630b-2a44-4167-8319-4873b4e3e0f0\"}]},\"type\":\"ConnectorPlacement.EquallySpacedConnector\",\"uuid\":\"48d452e0-ef32-4a0a-be11-1a1156200253\"}],\"packageUris\":[\"http://schema.mathworks.com/mf0/Connector/R2020b\"],\"version\":\"1.0\"}"
  Wrist1_Link : Subsystem
  Wrist2_Link : Subsystem
  base_link : Subsystem
  mount : Subsystem
  World : PMIOPort  Side=Left
  End Effector : PMIOPort  Port=2  Side=Right
  PV : Outport
  PD_torques : Outport  Port=2
  wires:
  Constant3/1 -> Simulink-PS Converter1/1
  Constant4/1 -> Simulink-PS Converter4/1
  torque/1 -> Demux1/1
  PSS11/1 -> Mux1/6  "V_R6"
  PSS8/1 -> Mux1/5  "P_R6"
  PSS5/1 -> Mux1/4  "V_R3"
  PSS4/1 -> Mux1/3  "P_R3"
  PSS3/1 -> Mux1/2  "V_R2"
  PSS2/1 -> Mux1/1  "P_R2"
  Mux1/1 -> PV/1
  PSS12/1 -> Mux1/7  "P_R7"
  PSS13/1 -> Mux1/8  "V_R7"
  PS-Simulink Converter1/1 -> Scope1/1
  Constant5/1 -> Simulink-PS Converter5/1
  PS-Simulink Converter2/1 -> Scope2/1
  Constant7/1 -> Simulink-PS Converter7/1
  PS-Simulink Converter3/1 -> Scope3/1
  Constant1/1 -> Simulink-PS Converter3/1
  R7_q0/1 -> Torque controller J7/1(q0)
  R3_q0/1 -> Torque controller J3/1(q0)
  R6_q0/1 -> Torque controller J6/1(q0)
  R2_q0/1 -> Torque controller J2/1(q0)
  Demux1/2 -> Torque controller J3/2(rl_t)
  Demux1/3 -> Torque controller J6/2(rl_t)
  Demux1/4 -> Torque controller J7/2(rl_t)
  Demux1/1 -> Torque controller J2/2(rl_t)
  Delta torque/1 -> MATLAB Function/3(delta_torque)
  Torque/1 -> MATLAB Function/2(torque)
  Clock/1 -> MATLAB Function/1(t)
  MATLAB Function/1(dummy) -> Terminator/1
  Torque controller J2/1(torque J2) -> PD torques/1
  Torque controller J3/2(torque J2) -> PD torques/2
  Torque controller J6/2(torque J6) -> PD torques/3
  Torque controller J7/2(torque J7) -> PD torques/4
  PD torques/1 -> PD_torques/1
  connections:
  Actuator1/RConn1 -- Shoulder_Link/LConn1
  Actuator2/RConn1 -- HalfArm1_Link/LConn1
  Actuator1/LConn1 -- base_link/RConn1
  Actuator7/LConn1 -- Wrist2_Link/RConn1
  Actuator3/RConn1 -- HalfArm2_Link/LConn1
  Actuator4/LConn1 -- HalfArm2_Link/RConn1
  Actuator6/LConn1 -- Wrist1_Link/RConn1
  Actuator4/RConn1 -- ForeArm_Link/LConn1
  Actuator3/LConn1 -- HalfArm1_Link/RConn1
  Bracelet_Link/RConn1 -- Endeffector/LConn1
  Actuator5/RConn1 -- Wrist1_Link/LConn1
  Actuator5/LConn1 -- ForeArm_Link/RConn1
  Actuator2/LConn1 -- Shoulder_Link/RConn1
  Actuator6/RConn1 -- Wrist2_Link/LConn1
  Actuator7/RConn1 -- Bracelet_Link/LConn1
  Simulink-PS Converter1/RConn1 -- Actuator4/LConn2
  End Effector/RConn1 -- EF Attachment/RConn1
  EF Attachment/LConn1 -- Endeffector/RConn1
  World/RConn1 -- mount/RConn1
  mount/LConn1 -- base_link/LConn1
  Actuator3/RConn2 -- PSS4/LConn1 -- Torque controller J3/RConn2
  Actuator3/RConn3 -- Torque controller J3/RConn1 -- PSS5/LConn1
  Actuator6/RConn2 -- Torque controller J6/RConn1 -- PSS8/LConn1
  Actuator6/RConn3 -- Torque controller J6/RConn3 -- PSS11/LConn1
  Actuator7/RConn2 -- Torque controller J7/RConn1 -- PSS12/LConn1
  Actuator7/RConn3 -- Torque controller J7/RConn2 -- PSS13/LConn1
  Simulink-PS Converter4/RConn1 -- Actuator5/LConn2
  Actuator2/RConn3 -- PSS3/LConn1 -- Torque controller J2/RConn2
  Actuator2/RConn2 -- Torque controller J2/RConn1 -- PSS2/LConn1
  Simulink-PS Converter3/RConn1 -- Actuator1/LConn2
  Actuator2/LConn2 -- Torque controller J2/RConn3
  Torque controller J3/RConn3 -- Actuator3/LConn2
  Torque controller J6/RConn2 -- Actuator6/LConn2
  Torque controller J7/RConn3 -- Actuator7/LConn2

== system rlKinovaBallBalance_lags/Kinova Ball Balance/Control ==
  Waypoints : Inport
  In Bus Element1 : Inport  Port=2  PortName=Rover  Element=Chassis
  In Bus Element5 : Inport  Port=2  PortName=Rover  Element=Body
  Chassis Control : Subsystem
  Out Bus Element1 : Outport  PortName=Ctrl  Element=Chassis
  wires:
  Waypoints/1 -> Chassis Control/1(Waypoints)
  Chassis Control/1(Ctrl) -> Out Bus Element1/1
  In Bus Element1/1 -> Chassis Control/2(Chassis)
  In Bus Element5/1 -> Chassis Control/3(Body)

== system rlKinovaBallBalance_lags/Kinova Ball Balance/Data2Fluent ==
  w_GVM : Inport
  v_GVM : Inport  Port=2
  q_GVM : Inport  Port=3
  p_GVM : Inport  Port=4
  isdone : Inport  Port=5
  Data Type Conversion : DataTypeConversion  OutDataTypeStr=double  SaturateOnIntegerOverflow=off  RndMeth=Floor
  Demux p : Demux  Outputs=3
  Demux q : Demux
  Demux v : Demux  Outputs=3
  Demux w : Demux  Outputs=3
  Mux : Mux  Inputs=14
  plate_data : Outport
  wires:
  q_GVM/1 -> Demux q/1
  Demux q/4 -> Mux/7  "q4"
  Demux p/1 -> Mux/1  "Px"
  Demux p/2 -> Mux/2  "Py"
  Demux p/3 -> Mux/3  "Pz"
  Demux q/1 -> Mux/4  "q1"
  Demux q/2 -> Mux/5  "q2"
  Demux q/3 -> Mux/6  "q3"
  Demux v/1 -> Mux/8  "vx"
  Demux v/2 -> Mux/9  "vy"
  Demux v/3 -> Mux/10  "vz"
  Mux/1 -> plate_data/1
  Demux w/1 -> Mux/11  "wx"
  Demux w/2 -> Mux/12  "wy"
  Demux w/3 -> Mux/13  "wz"
  isdone/1 -> Data Type Conversion/1
  Data Type Conversion/1 -> Mux/14
  v_GVM/1 -> Demux v/1
  w_GVM/1 -> Demux w/1
  p_GVM/1 -> Demux p/1

== system rlKinovaBallBalance_lags/Kinova Ball Balance/Done ==
  vol_spill : Inport
  liquid_mass : Inport  Port=2
  AND : Logic  IconShape=distinctive  AllPortsSameDT=off  OutDataTypeStr=boolean
  Compare To Constant : simulink/Logic and Bit Operations/Compare To Constant  relop=>  const=0  OutDataTypeStr=boolean
  Compare To Constant1 : simulink/Logic and Bit Operations/Compare To Constant  relop=<  const=fluent0.m*0.7  OutDataTypeStr=boolean
  Compare To Constant2 : simulink/Logic and Bit Operations/Compare To Constant  relop=>=  const=fluent0.m*0.3*0.001  OutDataTypeStr=boolean
  OR : Logic  Operator=OR  IconShape=distinctive  AllPortsSameDT=off  OutDataTypeStr=boolean
  done : Outport
  wires:
  AND/1 -> OR/2
  Compare To Constant1/1 -> AND/1
  Compare To Constant/1 -> AND/2
  liquid_mass/1 -> Compare To Constant/1, Compare To Constant1/1
  OR/1 -> done/1
  vol_spill/1 -> Compare To Constant2/1
  Compare To Constant2/1 -> OR/1

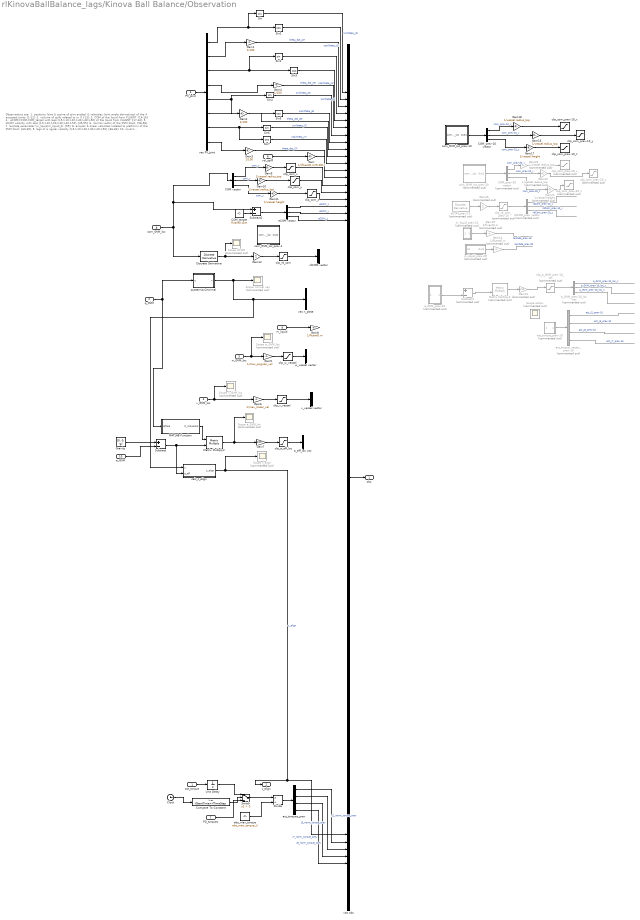
== system rlKinovaBallBalance_lags/Kinova Ball Balance/Observation ==
  note: Observations are:
      | 1. positions (sine & cosine of joint angles) & velocities (joint angle derivatives) of the 4 actuated joints {1-12}
      | 2. volume of spills related to m_0 {13}
      | 3. COM of the liquid from FLUENT {14-16}
      | 4 . eCOM=COM-COM_target with lags [t-5,t-10,t-20,t-30,t-40,t-50] of the liquid from FLUENT {17-34}
      | 5. dCOM velocity with lags [t-5,t-10,t-20,t-30,t-40,t-50] {35-55}
      | 6. normal vector of the GVM block {56-58}
      | 7. lambda parameter (m_liquid/m_liquid_0) {59}
      | 8. angular & linear velocities (related to platform) of the GVM block {60-65}
      | 9. lags of a ngular velocity [t-5,t-10,t-20,t-30,t-40,t-50] {66-83}
      | 10. rover's acceleration related to GVM local system a_eff_loc=quatToR_W2vessel[qPlate](Mars_gravity-a_chassis) {84-86}
      | 11. lags of a_eff_loc [t-5,t-10,t-20,t-30,t-40,t-50] {87-104}
      | 12. c_align = a_GVM / (||a_GVM||+epsilon)*dot*n_plate {105}
      | 13. 1-step lag for torques: act_torque_prev {106-109}
  act_torque : Inport
  q_GVM : Inport  Port=2
  PV_Joint : Inport  Port=3
  v_GVM_loc : Inport  Port=4
  w_GVM_loc : Inport  Port=5
  vol_spilll : Inport  Port=6
  PD_torques : Inport  Port=7
  com_GVM_loc : Inport  Port=8
  m_liquid : Inport  Port=9
  a_GVM : Inport  Port=10
  COM vector : Demux  Outputs=3
  COM_prev-10 vector : Demux  Outputs=3
  COM_prev-20 vector : Demux  Commented=on  Outputs=3
  COM_target : Constant  Value=fluent0.com
  Clock : Clock
  Compare To Constant : simulink/Logic and Bit Operations/Compare To Constant  relop=>=  const=rlStartTime+rlTimeStep  OutDataTypeStr=boolean
  Discrete Derivative : simulink/Discrete/Discrete Derivative  gainval=1.0  ICPrevScaledInput=0.0  OutMin=[]  OutMax=[]  OutDataType=fixdt(1, 16)  OutScaling=2^-10  DoSatur=off
  Divide : Product  Inputs=*/
  Gain : Gain  Gain=1/(fluent0.m*0.001)
  Gain{1..4} (4 alike) : Gain  Gain=1/100
  Gain{9..10,16,18} (4 alike) : Gain  Gain=1/vessel.radius_top
  Gain11 : Gain  Gain=1/vessel.height
  Gain12 : Gain
  Gain13 : Gain  Commented=on  Gain=1/10
  Gain14 : Gain  Commented=on  Gain=1/fluent0.m
  Gain15 : Gain  Commented=on
  Gain17 : Gain  Gain=1/vessel.height
  Gain19 : Gain  Commented=on  Gain=1/fluent0.m
  Gain20 : Gain  Commented=on  Gain=1/vessel.radius_top
  Gain21 : Gain  Commented=on  Gain=1/vessel.height
  Gain22 : Gain  Commented=on  Gain=1/vessel.radius_top
  Gain5 : Gain  Gain=1/max_angular_vel
  Gain6 : Gain  Gain=1/max_linear_vel
  Gain7 : Gain  Gain=1/10
  Gain8 : Gain  Gain=1/fluent0.m
  Gravity : Constant  Value=[0; 0; -g]
  MATLAB Function : MATLAB Function  TreatAsAtomicUnit=on
  Matrix Multiply2 : Product  Multiplication=Matrix(*)
  Matrix Multiply3 : Product  Commented=on  Multiplication=Matrix(*)
  Scope a_GVM_loc : Scope  Commented=on
  Scope action : Scope  Commented=on
  Scope c_align : Scope  Commented=on
  Scope dCOM : Scope  Commented=on
  Scope normal vec : Scope  Commented=on
  Scope v_GVM_loc : Scope  Commented=on
  Scope w_GVM_loc : Scope  Commented=on
  Sin{,1,4,6} (4 alike) : Trigonometry
  Sin{2..3,5,7} (4 alike) : Trigonometry  Operator=cos
  Subtract : Sum  Inputs=+-
  Subtract1 : Sum  Commented=on  Inputs=+-
  Subtract2 : Sum  Inputs=+-
  Switch : Switch  Criteria=u2 > Threshold  ZeroCross=off  SaturateOnIntegerOverflow=off  InputSameDT=off
  Unit Delay : UnitDelay  SampleTime=-1  HasFrameUpgradeWarning=on
  a_GVM_prev-10 : Subsystem  Commented=on
  a_GVM_prev-10_loc vec : Demux  Commented=on  Outputs=3
  a_eff_loc vec : Demux  Outputs=3
  abs_max_torque : Constant  Value=abs_max_torque_U
  act_torque_prev-10 : Subsystem  Commented=on
  act_torque_vector_prev-10 : Demux  Commented=on
  act_torques_prev : Demux
  calc_c_align : MATLAB Function  TreatAsAtomicUnit=on
  clip_a_GVM_prev-10_loc : Saturate  Commented=on  UpperLimit=1  LowerLimit=-1
  clip_a_eff_loc : Saturate  UpperLimit=1  LowerLimit=-1
  clip_com_prev-10_x : Saturate  UpperLimit=1  LowerLimit=-1
  clip_com_prev-10_y : Saturate  UpperLimit=1  LowerLimit=-1
  clip_com_prev-10_z : Saturate  UpperLimit=1  LowerLimit=-1
  clip_com_prev-20_x : Saturate  Commented=on  UpperLimit=1  LowerLimit=-1
  clip_com_prev-20_y : Saturate  Commented=on  UpperLimit=1  LowerLimit=-1
  clip_com_prev-20_z : Saturate  Commented=on  UpperLimit=1  LowerLimit=-1
  clip_com_x : Saturate  UpperLimit=1  LowerLimit=-1
  clip_com_y : Saturate  UpperLimit=1  LowerLimit=-1
  clip_com_z : Saturate  UpperLimit=1  LowerLimit=-1
  clip_rd_com : Saturate  UpperLimit=1  LowerLimit=-1
  clip_rd_com_prev-10 : Saturate  Commented=on  UpperLimit=1  LowerLimit=-1
  clip_v_vessel : Saturate  UpperLimit=1  LowerLimit=-1
  clip_w_vessel : Saturate  UpperLimit=1  LowerLimit=-1
  com_GVM_loc_prev-1 : Subsystem
  com_GVM_loc_prev-10 : Subsystem
  com_GVM_loc_prev-20 : Subsystem  Commented=on
  dCOM_prev-10 : simulink/Discrete/Discrete Derivative  Commented=on  gainval=1.0  ICPrevScaledInput=0.0  OutMin=[]  OutMax=[]  OutDataType=fixdt(1, 16)  OutScaling=2^-10  DoSatur=off
  eCOM vector : Demux  Outputs=3
  m_liquid_prev-10 : Subsystem  Commented=on
  m_liquid_prev-20 : Subsystem  Commented=on
  quaternion2normal : MATLAB Function  TreatAsAtomicUnit=on
  rdCOM vector : Demux  Outputs=3
  rdCOM_prev vector : Demux  Commented=on  Outputs=3
  v_vessel vector : Demux  Outputs=3
  vec PV_Joint : Demux  Outputs=8
  vec n_plate : Demux  Outputs=3
  vec obs : Mux  Inputs=109
  w_vessel vector : Demux  Outputs=3
  obs : Outport
  c_align : Outport  Port=2
  wires:
  PV_Joint/1 -> vec PV_Joint/1
  vec PV_Joint/1 -> Sin/1, Sin2/1
  vec PV_Joint/3 -> Sin1/1, Sin3/1
  vec PV_Joint/4 -> Gain4/1
  Sin/1 -> vec obs/1  "sin(theta_J2)"
  vec obs/1 -> obs/1
  Sin2/1 -> vec obs/2  "cos(theta_J2)"
  Sin1/1 -> vec obs/4  "sin(theta_J3)"
  Sin3/1 -> vec obs/5  "cos(theta_J3)"
  Gain1/1 -> vec obs/3  "theta_dot_J2*"
  vec PV_Joint/6 -> Gain2/1
  vec PV_Joint/8 -> Gain3/1
  Sin6/1 -> vec obs/10  "sin(theta_J7)"
  Sin7/1 -> vec obs/11  "cos(theta_J7)"
  Gain2/1 -> vec obs/9  "theta_dot_J6*"
  Gain3/1 -> vec obs/12  "theta_dot_J7*"
  COM vector/1 -> Gain9/1  "com_x"
  COM vector/2 -> Gain10/1  "com_y"
  COM vector/3 -> Gain11/1  "com_z"
  vol_spilll/1 -> Gain/1
  Gain/1 -> vec obs/13
  w_GVM_loc/1 -> Scope w_GVM_loc/1, Gain5/1
  v_GVM_loc/1 -> Scope v_GVM_loc/1, Gain6/1
  a_GVM/1 -> Subtract/2
  MATLAB Function/1(R_W2vessel) -> Matrix Multiply2/1
  Subtract/1 -> calc_c_align/2(a_eff), Matrix Multiply2/2
  Matrix Multiply2/1 -> Scope a_GVM_loc/1, Gain7/1
  Discrete Derivative/1 -> Scope dCOM/1, Gain12/1
  clip_rd_com/1 -> rdCOM vector/1
  Gain7/1 -> clip_a_eff_loc/1
  m_liquid/1 -> Gain8/1
  quaternion2normal/1(n) -> Scope normal vec/1, calc_c_align/1(n), vec n_plate/1
  q_GVM/1 -> quaternion2normal/1(q), MATLAB Function/1(qPlate)
  vec PV_Joint/7 -> Sin7/1, Sin6/1
  Sin4/1 -> vec obs/7  "sin(theta_J6)"
  Sin5/1 -> vec obs/8  "cos(theta_J6)"
  Gain4/1 -> vec obs/6  "theta_dot_J3*"
  vec PV_Joint/5 -> Sin5/1, Sin4/1
  Gain9/1 -> clip_com_x/1
  Gain11/1 -> clip_com_z/1
  Gain10/1 -> clip_com_y/1
  clip_com_x/1 -> vec obs/14
  clip_com_z/1 -> vec obs/16
  clip_com_y/1 -> vec obs/15
  Gain12/1 -> clip_rd_com/1
  calc_c_align/1(c_align) -> c_align/1, vec obs/105, Scope c_align/1  "c_align"
  Gravity/1 -> Subtract/1
  Gain5/1 -> clip_w_vessel/1
  clip_w_vessel/1 -> w_vessel vector/1
  Gain6/1 -> clip_v_vessel/1
  clip_v_vessel/1 -> v_vessel vector/1
  vec PV_Joint/2 -> Gain1/1
  clip_a_eff_loc/1 -> a_eff_loc vec/1
  COM_prev-10 vector/2 -> Gain16/1  "com_prev-10_y"
  Gain17/1 -> clip_com_prev-10_z/1
  COM_prev-10 vector/3 -> Gain17/1  "com_prev-10_z"
  Gain18/1 -> clip_com_prev-10_x/1
  com_GVM_loc_prev-10/1(Out1) -> COM_prev-10 vector/1
  Gain16/1 -> clip_com_prev-10_y/1
  COM_prev-10 vector/1 -> Gain18/1  "com_prev-10_x"
  COM_prev-20 vector/3 -> Gain21/1  "com_prev-20_z"
  COM_prev-20 vector/2 -> Gain20/1  "com_prev-20_y"
  COM_prev-20 vector/1 -> Gain22/1  "com_prev-20_x"
  Gain22/1 -> clip_com_prev-20_x/1
  Gain21/1 -> clip_com_prev-20_z/1
  Gain20/1 -> clip_com_prev-20_y/1
  com_GVM_loc_prev-20/1(Out1) -> COM_prev-20 vector/1
  Gain15/1 -> clip_rd_com_prev-10/1
  dCOM_prev-10/1 -> Gain15/1
  rdCOM_prev vector/1 -> ?  "rdCom_prev-10_x"
  rdCOM_prev vector/2 -> ?  "rdCom_prev-10_y"
  rdCOM_prev vector/3 -> ?  "rdCom_prev-10_z"
  clip_rd_com_prev-10/1 -> rdCOM_prev vector/1
  Gain14/1 -> ?  "lambda_prev-20"
  m_liquid_prev-10/1(Out1) -> Gain19/1
  Gain19/1 -> ?  "lambda_prev-10"
  m_liquid_prev-20/1(Out1) -> Gain14/1
  a_GVM_prev-10_loc vec/3 -> ?  "a_GVM_prev-10_loc_z"
  act_torque_prev-10/1(Out1) -> act_torque_vector_prev-10/1
  a_GVM_prev-10/1(Out1) -> Subtract1/2
  a_GVM_prev-10_loc vec/2 -> ?  "a_GVM_prev-10_loc_y"
  Gain13/1 -> clip_a_GVM_prev-10_loc/1
  act_torque_vector_prev-10/3 -> ?  "act_J6_prev-10"
  Matrix Multiply3/1 -> Gain13/1
  act_torque_vector_prev-10/4 -> ?  "act_J7_prev-10"
  Subtract1/1 -> Matrix Multiply3/2
  clip_a_GVM_prev-10_loc/1 -> a_GVM_prev-10_loc vec/1
  act_torque_vector_prev-10/2 -> ?  "act_J3_prev-10"
  a_GVM_prev-10_loc vec/1 -> ?  "a_GVM_prev-10_loc_x"
  act_torque_vector_prev-10/1 -> ?  "act_J2_prev-10"
  act_torques_prev/1 -> vec obs/106  "J2_norm_torque_prev"
  act_torques_prev/2 -> vec obs/107  "J3_norm_torque_prev"
  act_torques_prev/3 -> vec obs/108  "J6_norm_torque_prev"
  act_torques_prev/4 -> vec obs/109  "J7_norm_torque_prev"
  Divide/1 -> act_torques_prev/1
  abs_max_torque/1 -> Divide/2
  Clock/1 -> Compare To Constant/1
  Compare To Constant/1 -> Switch/2
  Switch/1 -> Divide/1
  act_torque/1 -> Unit Delay/1
  PD_torques/1 -> Switch/3
  Unit Delay/1 -> Switch/1
  Subtract2/1 -> eCOM vector/1
  com_GVM_loc/1 -> Subtract2/1, COM vector/1, Discrete Derivative/1
  COM_target/1 -> Subtract2/2
  eCOM vector/1 -> vec obs/17  "eCOM_x"
  eCOM vector/2 -> vec obs/18  "eCOM_y"
  eCOM vector/3 -> vec obs/19  "eCOM_z"
